simulink model "EGRVlv_VDMon_5818"  (R2016b)
settings: configuration reference "CodeGenConfigSet" (kept outside this file)
values from neighbouring files (symbols this model uses):
  EGRVlv_numLckdDetThres_C = Calibration.Parameter    [init_EGRVlv_VDMon.m]    (also in init_EGRVlv_VDMon_SIL.m = Simulink.Parameter)
  EGRVlv_numMonEngTemp_C = Calibration.Parameter    [init_EGRVlv_VDMon.m]    (also in init_EGRVlv_VDMon_SIL.m = Simulink.Parameter)
  EGRVlv_rDvtMax_C = Calibration.Parameter    [init_EGRVlv_VDMon.m]    (also in init_EGRVlv_VDMon_SIL.m = Simulink.Parameter)
  EGRVlv_rDvtMin_C = Calibration.Parameter    [init_EGRVlv_VDMon.m]    (also in init_EGRVlv_VDMon_SIL.m = Simulink.Parameter)
  EGRVlv_rJamVlvOpnDemMax_C = Calibration.Parameter    [init_EGRVlv_VDMon.m]    (also in init_EGRVlv_VDMon_SIL.m = Simulink.Parameter)
  EGRVlv_rJamVlvOpnHi_C = Calibration.Parameter    [init_EGRVlv_VDMon.m]    (also in init_EGRVlv_VDMon_SIL.m = Simulink.Parameter)
  EGRVlv_rJamVlvOpnLo_C = Calibration.Parameter    [init_EGRVlv_VDMon.m]    (also in init_EGRVlv_VDMon_SIL.m = Simulink.Parameter)
  EGRVlv_rLckdDetThres_C = Calibration.Parameter    [init_EGRVlv_VDMon.m]    (also in init_EGRVlv_VDMon_SIL.m = Simulink.Parameter)
  EGRVlv_rLMSActPosThresInit_C = Calibration.Parameter    [init_EGRVlv_VDMon.m]    (also in init_EGRVlv_VDMon_SIL.m = Simulink.Parameter)
  EGRVlv_rLMSActThresDwn_C = Calibration.Parameter    [init_EGRVlv_VDMon.m]    (also in init_EGRVlv_VDMon_SIL.m = Simulink.Parameter)
  EGRVlv_rLMSThresDwn_C = Calibration.Parameter    [init_EGRVlv_VDMon.m]    (also in init_EGRVlv_VDMon_SIL.m = Simulink.Parameter)
  EGRVlv_rLMSThresUp_C = Calibration.Parameter    [init_EGRVlv_VDMon.m]    (also in init_EGRVlv_VDMon_SIL.m = Simulink.Parameter)
  EGRVlv_RlsIKi_C = Calibration.Parameter    [init_EGRVlv_VDMon.m]    (also in init_EGRVlv_VDMon_SIL.m = Simulink.Parameter)
  EGRVlv_rRlsMax_C = Calibration.Parameter    [init_EGRVlv_VDMon.m]    (also in init_EGRVlv_VDMon_SIL.m = Simulink.Parameter)
  EGRVlv_rStpThres_C = Calibration.Parameter    [init_EGRVlv_VDMon.m]    (also in init_EGRVlv_VDMon_SIL.m = Simulink.Parameter)
  EGRVlv_swtGovByp_C = Calibration.Parameter    [init_EGRVlv_VDMon.m]    (also in init_EGRVlv_VDMon_SIL.m = Simulink.Parameter)
  EGRVlv_tEngHi_C = Calibration.Parameter    [init_EGRVlv_VDMon.m]    (also in init_EGRVlv_VDMon_SIL.m = Simulink.Parameter)
  EGRVlv_tEngLo_C = Calibration.Parameter    [init_EGRVlv_VDMon.m]    (also in init_EGRVlv_VDMon_SIL.m = Simulink.Parameter)
  EGRVlv_tiGovDvtMaxDebDef_C = Calibration.Parameter    [init_EGRVlv_VDMon.m]    (also in init_EGRVlv_VDMon_SIL.m = Simulink.Parameter)
  EGRVlv_tiGovDvtMaxDebOk_C = Calibration.Parameter    [init_EGRVlv_VDMon.m]    (also in init_EGRVlv_VDMon_SIL.m = Simulink.Parameter)
  EGRVlv_tiGovDvtMinDebDef_C = Calibration.Parameter    [init_EGRVlv_VDMon.m]    (also in init_EGRVlv_VDMon_SIL.m = Simulink.Parameter)
  EGRVlv_tiGovDvtMinDebOk_C = Calibration.Parameter    [init_EGRVlv_VDMon.m]    (also in init_EGRVlv_VDMon_SIL.m = Simulink.Parameter)
  EGRVlv_tiLMS_C = Calibration.Parameter    [init_EGRVlv_VDMon.m]    (also in init_EGRVlv_VDMon_SIL.m = Simulink.Parameter)
  EGRVlv_tiRepRls_C = Calibration.Parameter    [init_EGRVlv_VDMon.m]    (also in init_EGRVlv_VDMon_SIL.m = Simulink.Parameter)
  EGRVlv_tiRls_C = Calibration.Parameter    [init_EGRVlv_VDMon.m]    (also in init_EGRVlv_VDMon_SIL.m = Simulink.Parameter)
undefined symbols (not defined in the file or in its folder): EGRVlv_VDMon_DT, EngState_conv
libraries: CXLib x25, simulink x14
settings Model: Creator=lvzhanghui  LastModifiedBy=zhulinfeng
settings ConfigSetRef: SourceLocation=Base Workspace

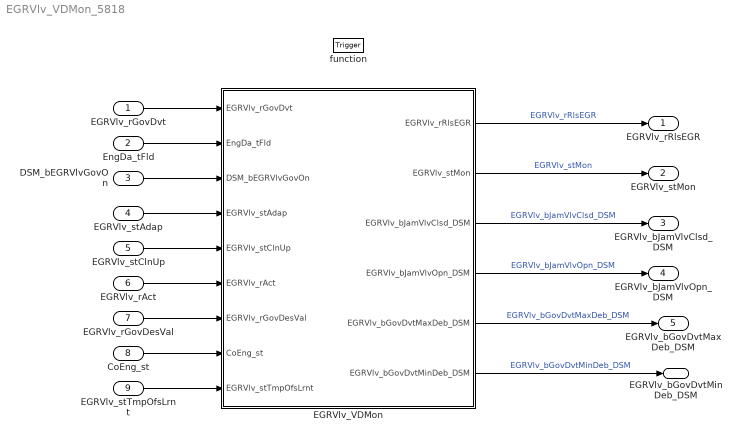
== system EGRVlv_VDMon_5818 ==
  EGRVlv_rGovDvt : Inport  Tag=%  Description=Control deviation  OutMin=-100  OutMax=100  OutDataTypeStr=Prc_100_rate
  EngDa_tFld : Inport  Tag=deg  Description=Engine temperature field  Port=2  OutMin=-3000  OutMax=3000  OutDataTypeStr=Temp_deg  PortDimensions=3
  DSM_bEGRVlvGovOn : Inport  Description=Status of FId_EGRVlvGovOn  Port=3  OutMin=0  OutMax=1  OutDataTypeStr=boolean
  EGRVlv_stAdap : Inport  Description=Status of offset learning  Port=4  OutMin=0  OutMax=65535  OutDataTypeStr=State_uint16
  EGRVlv_stClnUp : Inport  Description=Status of valvle cleanup function  Port=5  OutMin=0  OutMax=255  OutDataTypeStr=State_uint8
  EGRVlv_rAct : Inport  Tag=%  Description=Actuatorposition  Port=6  OutMin=-100  OutMax=100  OutDataTypeStr=Prc_100_rate
  EGRVlv_rGovDesVal : Inport  Tag=%  Description=Internal desired value for governor  Port=7  OutMin=-100  OutMax=100  OutDataTypeStr=Prc_100_rate
  CoEng_st : Inport  Description=Engine coordinator state  Port=8  OutDataTypeStr=Enum: EngState_conv
  EGRVlv_stTmpOfsLrnt : Inport  Description=Temporary offset of the EGR valve is already learnt in the current driving cycle  Port=9  OutMin=0  OutMax=1  OutDataTypeStr=boolean
  function : TriggerPort  TriggerType=function-call  VariantControl=Variant
  EGRVlv_VDMon : Subsystem
  EGRVlv_rRlsEGR : Outport  Tag=%  Description=Additional control value to release a jammed valve  OutMin=-100  OutMax=100  OutDataTypeStr=Prc_100_rate
  EGRVlv_stMon : Outport  Description=State of system monitoring  Port=2  OutMin=0  OutMax=65535  OutDataTypeStr=State_uint16
  EGRVlv_bJamVlvClsd_DSM : Outport  Description=Status of EGRVlv_bJamVlvClsd  Port=3  OutMin=0  OutMax=1  OutDataTypeStr=boolean
  EGRVlv_bJamVlvOpn_DSM : Outport  Description=Status of EGRVlv_bJamVlvOpn  Port=4  OutMin=0  OutMax=1  OutDataTypeStr=boolean
  EGRVlv_bGovDvtMaxDeb_DSM : Outport  Description=Status of EGRVlv_bGovDvtMaxDeb  Port=5  OutMin=0  OutMax=1  OutDataTypeStr=boolean
  EGRVlv_bGovDvtMinDeb_DSM : Outport  Description=Status of EGRVlv_bGovDvtMinDeb  Port=6  OutMin=0  OutMax=1  OutDataTypeStr=boolean
  wires:
  EGRVlv_rGovDvt/1 -> EGRVlv_VDMon/1(EGRVlv_rGovDvt)
  EngDa_tFld/1 -> EGRVlv_VDMon/2(EngDa_tFld)
  DSM_bEGRVlvGovOn/1 -> EGRVlv_VDMon/3(DSM_bEGRVlvGovOn)
  EGRVlv_stAdap/1 -> EGRVlv_VDMon/4(EGRVlv_stAdap)
  EGRVlv_stClnUp/1 -> EGRVlv_VDMon/5(EGRVlv_stClnUp)
  EGRVlv_rAct/1 -> EGRVlv_VDMon/6(EGRVlv_rAct)
  EGRVlv_rGovDesVal/1 -> EGRVlv_VDMon/7(EGRVlv_rGovDesVal)
  CoEng_st/1 -> EGRVlv_VDMon/8(CoEng_st)
  EGRVlv_stTmpOfsLrnt/1 -> EGRVlv_VDMon/9(EGRVlv_stTmpOfsLrnt)
  EGRVlv_VDMon/1(EGRVlv_rRlsEGR) -> EGRVlv_rRlsEGR/1  "EGRVlv_rRlsEGR"
  EGRVlv_VDMon/2(EGRVlv_stMon) -> EGRVlv_stMon/1  "EGRVlv_stMon"
  EGRVlv_VDMon/3(EGRVlv_bJamVlvClsd_DSM) -> EGRVlv_bJamVlvClsd_DSM/1  "EGRVlv_bJamVlvClsd_DSM"
  EGRVlv_VDMon/4(EGRVlv_bJamVlvOpn_DSM) -> EGRVlv_bJamVlvOpn_DSM/1  "EGRVlv_bJamVlvOpn_DSM"
  EGRVlv_VDMon/6(EGRVlv_bGovDvtMinDeb_DSM) -> EGRVlv_bGovDvtMinDeb_DSM/1  "EGRVlv_bGovDvtMinDeb_DSM"
  EGRVlv_VDMon/5(EGRVlv_bGovDvtMaxDeb_DSM) -> EGRVlv_bGovDvtMaxDeb_DSM/1  "EGRVlv_bGovDvtMaxDeb_DSM"

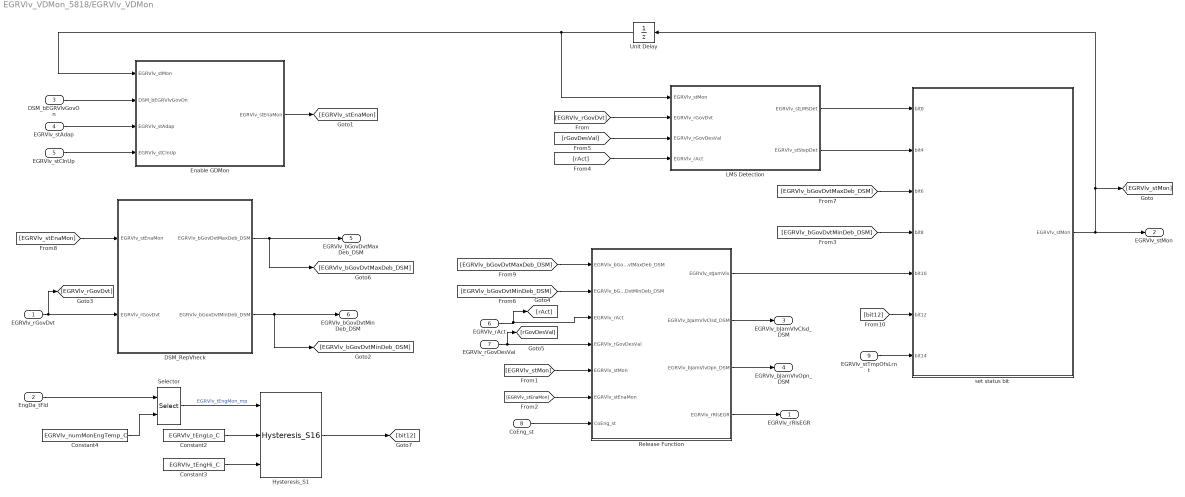
== system EGRVlv_VDMon_5818/EGRVlv_VDMon ==
  EGRVlv_rGovDvt : Inport  Tag=%
  EngDa_tFld : Inport  Tag=%  Port=2
  DSM_bEGRVlvGovOn : Inport  Tag=%  Port=3
  EGRVlv_stAdap : Inport  Tag=%  Port=4
  EGRVlv_stClnUp : Inport  Tag=%  Port=5
  EGRVlv_rAct : Inport  Tag=%  Port=6
  EGRVlv_rGovDesVal : Inport  Tag=%  Port=7
  CoEng_st : Inport  Tag=%  Port=8
  EGRVlv_stTmpOfsLrnt : Inport  Tag=%  Port=9
  Constant2 : Constant  Value=EGRVlv_tEngLo_C  SampleTime=-1
  Constant3 : Constant  Value=EGRVlv_tEngHi_C  SampleTime=-1
  Constant4 : Constant  Value=EGRVlv_numMonEngTemp_C  SampleTime=-1
  DSM_RepVheck : Subsystem
  Enable GDMon : Subsystem
  Hysteresis_S1 : CXLib/Hysteresis_S16
  LMS Detection : Subsystem
  Release Function : Subsystem
  Selector : Selector  IndexMode=Zero-based  InputPortWidth=3  IndexOptions=Index vector (port)  Indices=[1 3]  OutputSizes=1
  Unit Delay : UnitDelay  SampleTime=-1
      settings: AttributesFormatString=InitialValue=%<InitialCondition>
  set status bit : Subsystem
  EGRVlv_rRlsEGR : Outport  Tag=%
  EGRVlv_stMon : Outport  Tag=%  Port=2
  EGRVlv_bJamVlvClsd_DSM : Outport  Tag=%  Port=3
  EGRVlv_bJamVlvOpn_DSM : Outport  Tag=%  Port=4
  EGRVlv_bGovDvtMaxDeb_DSM : Outport  Description=Status of EGRVlv_bGovDvtMaxDeb  Port=5  OutMin=0  OutMax=1  OutDataTypeStr=boolean
  EGRVlv_bGovDvtMinDeb_DSM : Outport  Description=Status of EGRVlv_bGovDvtMinDeb  Port=6  OutMin=0  OutMax=1  OutDataTypeStr=boolean
  wires:
  Selector/1 -> Hysteresis_S1/1  "EGRVlv_tEngMon_mp"
  Release Function/1(EGRVlv_stJamVlv) -> set status bit/5(bit10)
  set status bit/1(EGRVlv_stMon) -> Unit Delay/1, [EGRVlv_stMon], EGRVlv_stMon/1
  Constant2/1 -> Hysteresis_S1/2
  DSM_RepVheck/2(EGRVlv_bGovDvtMinDeb_DSM) -> [EGRVlv_bGovDvtMinDeb_DSM], EGRVlv_bGovDvtMinDeb_DSM/1
  Constant3/1 -> Hysteresis_S1/3
  DSM_RepVheck/1(EGRVlv_bGovDvtMaxDeb_DSM) -> [EGRVlv_bGovDvtMaxDeb_DSM], EGRVlv_bGovDvtMaxDeb_DSM/1
  Constant4/1 -> Selector/2
  EngDa_tFld/1 -> Selector/1
  EGRVlv_rGovDvt/1 -> [EGRVlv_rGovDvt], DSM_RepVheck/2(EGRVlv_rGovDvt)
  EGRVlv_rAct/1 -> [rAct], Release Function/3(EGRVlv_rAct)
  EGRVlv_rGovDesVal/1 -> [rGovDesVal], Release Function/4(EGRVlv_rGovDesVal)
  Unit Delay/1 -> Enable GDMon/1(EGRVlv_stMon), LMS Detection/1(EGRVlv_stMon)
  LMS Detection/2(EGRVlv_stStepDet) -> set status bit/2(bit4)
  LMS Detection/1(EGRVlv_stLMSDet) -> set status bit/1(bit0)
  Enable GDMon/1(EGRVlv_stEnaMon) -> [EGRVlv_stEnaMon]
  DSM_bEGRVlvGovOn/1 -> Enable GDMon/2(DSM_bEGRVlvGovOn)
  EGRVlv_stAdap/1 -> Enable GDMon/3(EGRVlv_stAdap)
  EGRVlv_stClnUp/1 -> Enable GDMon/4(EGRVlv_stClnUp)
  [EGRVlv_rGovDvt] -> LMS Detection/2(EGRVlv_rGovDvt)
  [rGovDesVal] -> LMS Detection/3(EGRVlv_rGovDesVal)
  [rAct] -> LMS Detection/4(EGRVlv_rAct)
  [EGRVlv_stMon] -> Release Function/5(EGRVlv_stMon)
  [EGRVlv_stEnaMon] -> Release Function/6(EGRVlv_stEnaMon)
  CoEng_st/1 -> Release Function/7(CoEng_st)
  [EGRVlv_bGovDvtMinDeb_DSM] -> set status bit/4(bit8)
  EGRVlv_stTmpOfsLrnt/1 -> set status bit/7(bit14)
  Release Function/2(EGRVlv_bJamVlvClsd_DSM) -> EGRVlv_bJamVlvClsd_DSM/1
  Release Function/3(EGRVlv_bJamVlvOpn_DSM) -> EGRVlv_bJamVlvOpn_DSM/1
  Release Function/4(EGRVlv_rRlsEGR) -> EGRVlv_rRlsEGR/1
  [EGRVlv_bGovDvtMinDeb_DSM] -> Release Function/2(EGRVlv_bGovDvtMinDeb_DSM)
  [EGRVlv_bGovDvtMaxDeb_DSM] -> set status bit/3(bit6)
  [EGRVlv_stEnaMon] -> DSM_RepVheck/1(EGRVlv_stEnaMon)
  [EGRVlv_bGovDvtMaxDeb_DSM] -> Release Function/1(EGRVlv_bGovDvtMaxDeb_DSM)
  Hysteresis_S1/1 -> [bit12]
  [bit12] -> set status bit/6(bit12)

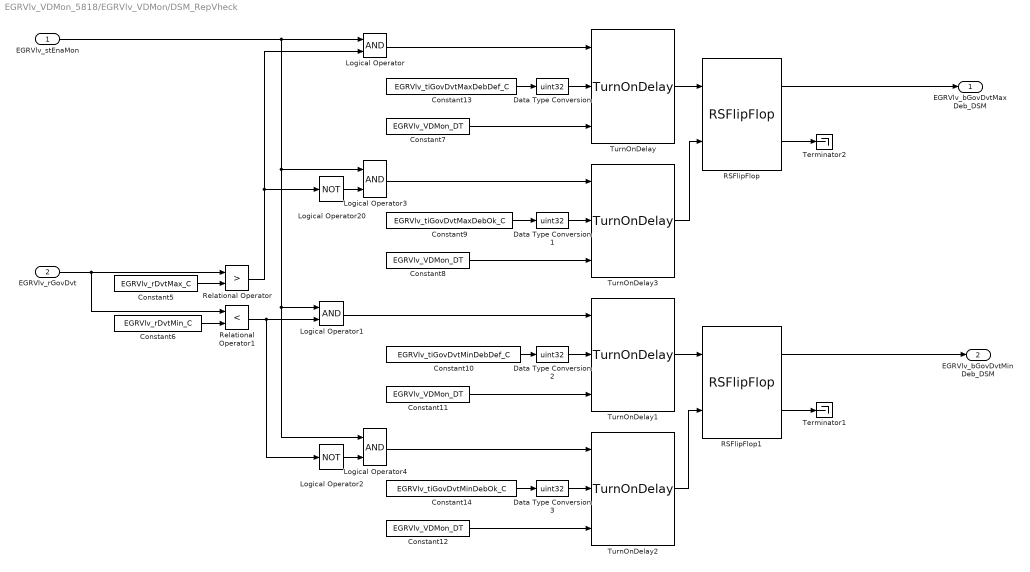
== system EGRVlv_VDMon_5818/EGRVlv_VDMon/DSM_RepVheck ==
  EGRVlv_stEnaMon : Inport  Tag=%
  EGRVlv_rGovDvt : Inport  Tag=%  Port=2
  Constant10 : Constant  Value=EGRVlv_tiGovDvtMinDebDef_C
  Constant{7..8,11..12} (4 alike) : Constant  Value=EGRVlv_VDMon_DT
  Constant13 : Constant  Value=EGRVlv_tiGovDvtMaxDebDef_C
  Constant14 : Constant  Value=EGRVlv_tiGovDvtMinDebOk_C
  Constant5 : Constant  Value=EGRVlv_rDvtMax_C  SampleTime=-1
  Constant6 : Constant  Value=EGRVlv_rDvtMin_C  SampleTime=-1
  Constant9 : Constant  Value=EGRVlv_tiGovDvtMaxDebOk_C
  Data Type Conversion{,1..3} (4 alike) : DataTypeConversion  OutDataTypeStr=uint32
  Logical Operator{,1,3..4} (4 alike) : Logic  AllPortsSameDT=off  OutDataTypeStr=boolean
  Logical Operator2 : Logic  Operator=NOT  AllPortsSameDT=off  OutDataTypeStr=boolean
  Logical Operator20 : Logic  Operator=NOT  AllPortsSameDT=off  OutDataTypeStr=boolean
  RSFlipFlop : CXLib/RSFlipFlop
  RSFlipFlop1 : CXLib/RSFlipFlop
  Relational Operator : RelationalOperator  Operator=>  OutDataTypeStr=boolean  RndMeth=Simplest
  Relational Operator1 : RelationalOperator  Operator=<  OutDataTypeStr=boolean  RndMeth=Simplest
  Terminator1 : Terminator
  Terminator2 : Terminator
  TurnOnDelay{,1..3} (4 alike) : CXLib/TurnOnDelay
  EGRVlv_bGovDvtMaxDeb_DSM : Outport  Tag=%
  EGRVlv_bGovDvtMinDeb_DSM : Outport  Tag=%  Port=2
  wires:
  Constant9/1 -> Data Type Conversion1/1
  Constant12/1 -> TurnOnDelay2/3
  Logical Operator/1 -> TurnOnDelay/1
  Constant10/1 -> Data Type Conversion2/1
  TurnOnDelay2/1 -> RSFlipFlop1/2
  TurnOnDelay1/1 -> RSFlipFlop1/1
  Constant8/1 -> TurnOnDelay3/3
  Relational Operator1/1 -> Logical Operator2/1, Logical Operator1/2
  Constant11/1 -> TurnOnDelay1/3
  EGRVlv_rGovDvt/1 -> Relational Operator/1, Relational Operator1/1
  Relational Operator/1 -> Logical Operator/2, Logical Operator20/1
  Constant6/1 -> Relational Operator1/2
  Logical Operator1/1 -> TurnOnDelay1/1
  Constant13/1 -> Data Type Conversion/1
  TurnOnDelay3/1 -> RSFlipFlop/2
  Constant7/1 -> TurnOnDelay/3
  Constant14/1 -> Data Type Conversion3/1
  Constant5/1 -> Relational Operator/2
  TurnOnDelay/1 -> RSFlipFlop/1
  EGRVlv_stEnaMon/1 -> Logical Operator3/1, Logical Operator4/1, Logical Operator1/1, Logical Operator/1
  Data Type Conversion/1 -> TurnOnDelay/2
  Data Type Conversion1/1 -> TurnOnDelay3/2
  Data Type Conversion2/1 -> TurnOnDelay1/2
  Data Type Conversion3/1 -> TurnOnDelay2/2
  Logical Operator20/1 -> Logical Operator3/2
  Logical Operator3/1 -> TurnOnDelay3/1
  Logical Operator2/1 -> Logical Operator4/2
  Logical Operator4/1 -> TurnOnDelay2/1
  RSFlipFlop1/1 -> EGRVlv_bGovDvtMinDeb_DSM/1
  RSFlipFlop1/2 -> Terminator1/1
  RSFlipFlop/1 -> EGRVlv_bGovDvtMaxDeb_DSM/1
  RSFlipFlop/2 -> Terminator2/1

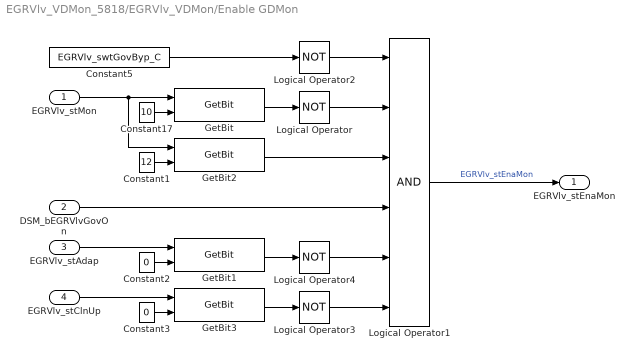
== system EGRVlv_VDMon_5818/EGRVlv_VDMon/Enable GDMon ==
  EGRVlv_stMon : Inport  Tag=%
  DSM_bEGRVlvGovOn : Inport  Tag=%  Port=2
  EGRVlv_stAdap : Inport  Tag=%  Port=3
  EGRVlv_stClnUp : Inport  Tag=%  Port=4
  Constant1 : Constant  Value=12  OutDataTypeStr=uint8
  Constant17 : Constant  Value=10  OutDataTypeStr=uint8
  Constant2 : Constant  Value=0  OutDataTypeStr=uint8
  Constant3 : Constant  Value=0  OutDataTypeStr=uint8
  Constant5 : Constant  Value=EGRVlv_swtGovByp_C  SampleTime=-1
  GetBit : CXLib/GetBit  dataTypeString=uint16  dataLength=0
      settings: AttributesFormatString=Get bit from %<dataTypeString>
  GetBit1 : CXLib/GetBit  dataTypeString=uint16  dataLength=0
      settings: AttributesFormatString=Get bit from %<dataTypeString>
  GetBit2 : CXLib/GetBit  dataTypeString=uint16  dataLength=0
      settings: AttributesFormatString=Get bit from %<dataTypeString>
  GetBit3 : CXLib/GetBit  dataTypeString=uint8  dataLength=0
      settings: AttributesFormatString=Get bit from %<dataTypeString>
  Logical Operator{,2..4} (4 alike) : Logic  Operator=NOT  AllPortsSameDT=off  OutDataTypeStr=boolean
  Logical Operator1 : Logic  Inputs=6  AllPortsSameDT=off  OutDataTypeStr=boolean
  EGRVlv_stEnaMon : Outport  Tag=%
  wires:
  Logical Operator/1 -> Logical Operator1/2
  Constant5/1 -> Logical Operator2/1
  GetBit2/1 -> Logical Operator1/3
  GetBit1/1 -> Logical Operator4/1
  Logical Operator3/1 -> Logical Operator1/6
  GetBit3/1 -> Logical Operator3/1
  Logical Operator4/1 -> Logical Operator1/5
  Logical Operator1/1 -> EGRVlv_stEnaMon/1  "EGRVlv_stEnaMon"
  Logical Operator2/1 -> Logical Operator1/1
  DSM_bEGRVlvGovOn/1 -> Logical Operator1/4
  GetBit/1 -> Logical Operator/1
  Constant17/1 -> GetBit/2
  Constant1/1 -> GetBit2/2
  Constant2/1 -> GetBit1/2
  Constant3/1 -> GetBit3/2
  EGRVlv_stMon/1 -> GetBit2/1, GetBit/1
  EGRVlv_stAdap/1 -> GetBit1/1
  EGRVlv_stClnUp/1 -> GetBit3/1

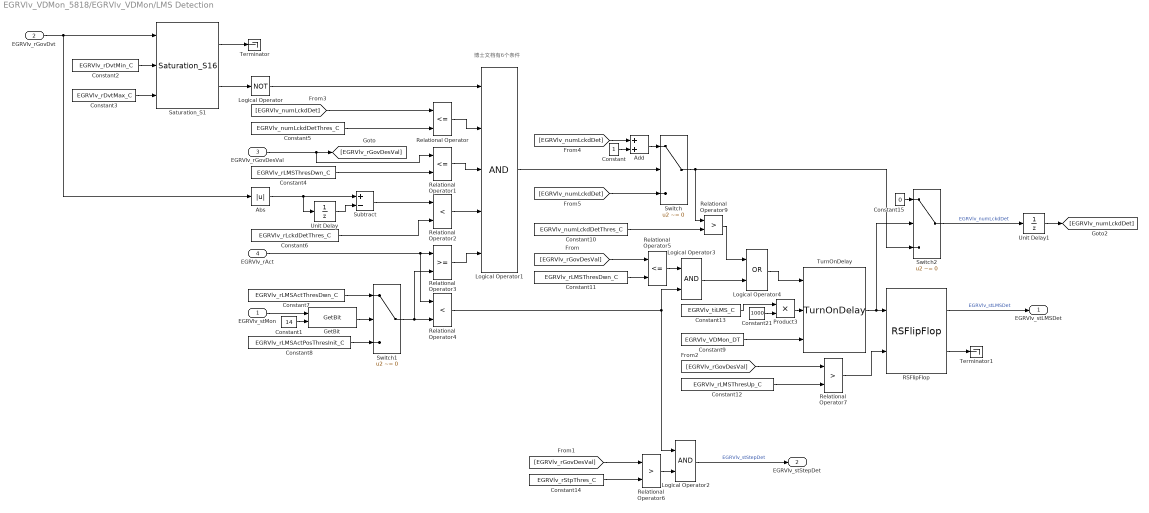
== system EGRVlv_VDMon_5818/EGRVlv_VDMon/LMS Detection ==
  note: 博士文档有6个条件
  EGRVlv_stMon : Inport  Tag=%
  EGRVlv_rGovDvt : Inport  Tag=%  Port=2
  EGRVlv_rGovDesVal : Inport  Tag=%  Port=3
  EGRVlv_rAct : Inport  Tag=%  Port=4
  Abs : Abs
  Add : Sum  SaturateOnIntegerOverflow=on
  Constant : Constant  OutDataTypeStr=Inherit: Inherit via back propagation
  Constant1 : Constant  Value=14  OutDataTypeStr=uint8
  Constant10 : Constant  Value=EGRVlv_numLckdDetThres_C
  Constant11 : Constant  Value=EGRVlv_rLMSThresDwn_C
  Constant12 : Constant  Value=EGRVlv_rLMSThresUp_C
  Constant13 : Constant  Value=EGRVlv_tiLMS_C
  Constant14 : Constant  Value=EGRVlv_rStpThres_C
  Constant15 : Constant  Value=0  OutDataTypeStr=Inherit: Inherit via back propagation
  Constant2 : Constant  Value=EGRVlv_rDvtMin_C  SampleTime=-1
  Constant21 : Constant  Value=1000  OutDataTypeStr=uint16
  Constant3 : Constant  Value=EGRVlv_rDvtMax_C  SampleTime=-1
  Constant4 : Constant  Value=EGRVlv_rLMSThresDwn_C  SampleTime=-1
  Constant5 : Constant  Value=EGRVlv_numLckdDetThres_C  SampleTime=-1
  Constant6 : Constant  Value=EGRVlv_rLckdDetThres_C  SampleTime=-1
  Constant7 : Constant  Value=EGRVlv_rLMSActThresDwn_C  SampleTime=-1
  Constant8 : Constant  Value=EGRVlv_rLMSActPosThresInit_C  SampleTime=-1
  Constant9 : Constant  Value=EGRVlv_VDMon_DT
  GetBit : CXLib/GetBit  dataTypeString=uint16  dataLength=0
      settings: AttributesFormatString=Get bit from %<dataTypeString>
  Logical Operator : Logic  Operator=NOT  AllPortsSameDT=off  OutDataTypeStr=boolean
  Logical Operator1 : Logic  Inputs=5  AllPortsSameDT=off  OutDataTypeStr=boolean
  Logical Operator2 : Logic  AllPortsSameDT=off  OutDataTypeStr=boolean
  Logical Operator3 : Logic  AllPortsSameDT=off  OutDataTypeStr=boolean
  Logical Operator4 : Logic  Operator=OR  AllPortsSameDT=off  OutDataTypeStr=boolean
  Product3 : Product  OutDataTypeStr=uint32  SaturateOnIntegerOverflow=on
  RSFlipFlop : CXLib/RSFlipFlop
  Relational Operator : RelationalOperator  Operator=<=  OutDataTypeStr=boolean  RndMeth=Simplest
  Relational Operator1 : RelationalOperator  Operator=<=  OutDataTypeStr=boolean  RndMeth=Simplest
  Relational Operator2 : RelationalOperator  Operator=<  OutDataTypeStr=boolean  RndMeth=Simplest
  Relational Operator3 : RelationalOperator  OutDataTypeStr=boolean  RndMeth=Simplest
  Relational Operator4 : RelationalOperator  Operator=<  OutDataTypeStr=boolean  RndMeth=Simplest
  Relational Operator5 : RelationalOperator  Operator=<=  OutDataTypeStr=boolean  RndMeth=Simplest
  Relational Operator6 : RelationalOperator  Operator=>  OutDataTypeStr=boolean  RndMeth=Simplest
  Relational Operator7 : RelationalOperator  Operator=>  OutDataTypeStr=boolean  RndMeth=Simplest
  Relational Operator9 : RelationalOperator  Operator=>  OutDataTypeStr=boolean  RndMeth=Simplest
  Saturation_S1 : CXLib/Saturation_S16
  Subtract : Sum  Inputs=+-  SaturateOnIntegerOverflow=on
  Switch : Switch  Criteria=u2 ~= 0
  Switch1 : Switch  Criteria=u2 ~= 0
  Switch2 : Switch  Criteria=u2 ~= 0
  Terminator : Terminator
  Terminator1 : Terminator
  TurnOnDelay : CXLib/TurnOnDelay
  Unit Delay : UnitDelay  SampleTime=-1
      settings: AttributesFormatString=InitialValue=%<InitialCondition>
  Unit Delay1 : UnitDelay  SampleTime=-1
      settings: AttributesFormatString=InitialValue=%<InitialCondition>
  EGRVlv_stLMSDet : Outport  Tag=%
  EGRVlv_stStepDet : Outport  Tag=%  Port=2
  wires:
  Saturation_S1/2 -> Logical Operator/1
  Constant1/1 -> GetBit/2
  Relational Operator/1 -> Logical Operator1/2
  Relational Operator1/1 -> Logical Operator1/3
  Relational Operator2/1 -> Logical Operator1/4
  Relational Operator3/1 -> Logical Operator1/5
  Constant5/1 -> Relational Operator/2
  Constant2/1 -> Saturation_S1/2
  Constant3/1 -> Saturation_S1/3
  EGRVlv_rGovDvt/1 -> Saturation_S1/1, Abs/1
  [EGRVlv_numLckdDet] -> Relational Operator/1
  Constant4/1 -> Relational Operator1/2
  EGRVlv_rGovDesVal/1 -> [EGRVlv_rGovDesVal], Relational Operator1/1
  Subtract/1 -> Relational Operator2/1
  Abs/1 -> Unit Delay/1, Subtract/1
  Unit Delay/1 -> Subtract/2
  Constant6/1 -> Relational Operator2/2
  Logical Operator1/1 -> Switch/2
  Add/1 -> Switch/1
  Constant/1 -> Add/2
  Constant7/1 -> Switch1/1
  Constant8/1 -> Switch1/3
  GetBit/1 -> Switch1/2
  Switch1/1 -> Relational Operator3/2, Relational Operator4/2
  Relational Operator6/1 -> Logical Operator2/2
  Relational Operator4/1 -> Logical Operator2/1, Logical Operator3/2
  Relational Operator5/1 -> Logical Operator3/1
  Logical Operator3/1 -> Logical Operator4/2
  Relational Operator9/1 -> Logical Operator4/1
  Constant9/1 -> TurnOnDelay/3
  TurnOnDelay/1 -> RSFlipFlop/1, Switch2/2
  Logical Operator4/1 -> TurnOnDelay/1
  Relational Operator7/1 -> RSFlipFlop/2
  Constant10/1 -> Relational Operator9/2
  [EGRVlv_rGovDesVal] -> Relational Operator5/1
  Constant11/1 -> Relational Operator5/2
  Constant12/1 -> Relational Operator7/2
  Constant14/1 -> Relational Operator6/2
  [EGRVlv_rGovDesVal] -> Relational Operator7/1
  Logical Operator2/1 -> EGRVlv_stStepDet/1  "EGRVlv_stStepDet"
  EGRVlv_rAct/1 -> Relational Operator4/1, Relational Operator3/1
  Constant15/1 -> Switch2/1
  Switch2/1 -> Unit Delay1/1  "EGRVlv_numLckdDet"
  Unit Delay1/1 -> [EGRVlv_numLckdDet]
  [EGRVlv_numLckdDet] -> Add/1
  [EGRVlv_numLckdDet] -> Switch/3
  Switch/1 -> Relational Operator9/1, Switch2/3
  [EGRVlv_rGovDesVal] -> Relational Operator6/1
  Logical Operator/1 -> Logical Operator1/1
  Constant21/1 -> Product3/2
  Constant13/1 -> Product3/1
  Product3/1 -> TurnOnDelay/2
  EGRVlv_stMon/1 -> GetBit/1
  RSFlipFlop/1 -> EGRVlv_stLMSDet/1  "EGRVlv_stLMSDet"
  RSFlipFlop/2 -> Terminator1/1
  Saturation_S1/1 -> Terminator/1

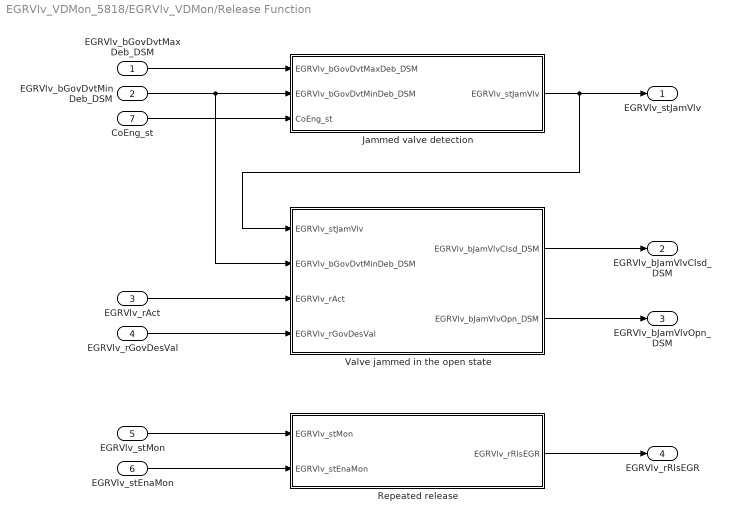
== system EGRVlv_VDMon_5818/EGRVlv_VDMon/Release Function ==
  EGRVlv_bGovDvtMaxDeb_DSM : Inport  Tag=%
  EGRVlv_bGovDvtMinDeb_DSM : Inport  Tag=%  Port=2
  EGRVlv_rAct : Inport  Tag=%  Port=3
  EGRVlv_rGovDesVal : Inport  Tag=%  Port=4
  EGRVlv_stMon : Inport  Tag=%  Port=5
  EGRVlv_stEnaMon : Inport  Tag=%  Port=6
  CoEng_st : Inport  Tag=%  Port=7
  Jammed valve detection : Subsystem
  Repeated release : Subsystem
  Valve jammed in the open state : Subsystem
  EGRVlv_stJamVlv : Outport  Tag=%
  EGRVlv_bJamVlvClsd_DSM : Outport  Tag=%  Port=2
  EGRVlv_bJamVlvOpn_DSM : Outport  Tag=%  Port=3
  EGRVlv_rRlsEGR : Outport  Tag=%  Port=4
  wires:
  EGRVlv_bGovDvtMinDeb_DSM/1 -> Jammed valve detection/2(EGRVlv_bGovDvtMinDeb_DSM), Valve jammed in the open state/2(EGRVlv_bGovDvtMinDeb_DSM)
  Jammed valve detection/1(EGRVlv_stJamVlv) -> EGRVlv_stJamVlv/1, Valve jammed in the open state/1(EGRVlv_stJamVlv)
  EGRVlv_bGovDvtMaxDeb_DSM/1 -> Jammed valve detection/1(EGRVlv_bGovDvtMaxDeb_DSM)
  CoEng_st/1 -> Jammed valve detection/3(CoEng_st)
  EGRVlv_stMon/1 -> Repeated release/1(EGRVlv_stMon)
  EGRVlv_stEnaMon/1 -> Repeated release/2(EGRVlv_stEnaMon)
  EGRVlv_rAct/1 -> Valve jammed in the open state/3(EGRVlv_rAct)
  EGRVlv_rGovDesVal/1 -> Valve jammed in the open state/4(EGRVlv_rGovDesVal)
  Repeated release/1(EGRVlv_rRlsEGR) -> EGRVlv_rRlsEGR/1
  Valve jammed in the open state/1(EGRVlv_bJamVlvClsd_DSM) -> EGRVlv_bJamVlvClsd_DSM/1
  Valve jammed in the open state/2(EGRVlv_bJamVlvOpn_DSM) -> EGRVlv_bJamVlvOpn_DSM/1

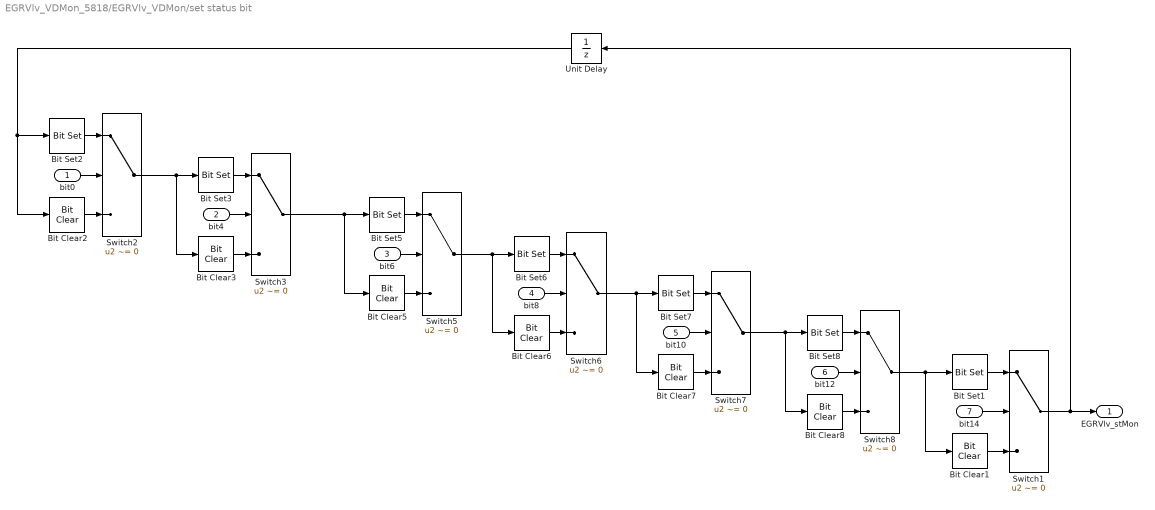
== system EGRVlv_VDMon_5818/EGRVlv_VDMon/set status bit ==
  bit0 : Inport
  bit4 : Inport  Port=2
  bit6 : Inport  Port=3
  bit8 : Inport  Port=4
  bit10 : Inport  Port=5
  bit12 : Inport  Port=6
  bit14 : Inport  Port=7
  Bit Clear1 : simulink/Logic and Bit Operations/Bit Clear  iBit=14
  Bit Clear2 : simulink/Logic and Bit Operations/Bit Clear  iBit=0
  Bit Clear3 : simulink/Logic and Bit Operations/Bit Clear  iBit=4
  Bit Clear5 : simulink/Logic and Bit Operations/Bit Clear  iBit=6
  Bit Clear6 : simulink/Logic and Bit Operations/Bit Clear  iBit=8
  Bit Clear7 : simulink/Logic and Bit Operations/Bit Clear  iBit=10
  Bit Clear8 : simulink/Logic and Bit Operations/Bit Clear  iBit=12
  Bit Set1 : simulink/Logic and Bit Operations/Bit Set  iBit=14
  Bit Set2 : simulink/Logic and Bit Operations/Bit Set  iBit=0
  Bit Set3 : simulink/Logic and Bit Operations/Bit Set  iBit=4
  Bit Set5 : simulink/Logic and Bit Operations/Bit Set  iBit=6
  Bit Set6 : simulink/Logic and Bit Operations/Bit Set  iBit=8
  Bit Set7 : simulink/Logic and Bit Operations/Bit Set  iBit=10
  Bit Set8 : simulink/Logic and Bit Operations/Bit Set  iBit=12
  Switch{1..3,5..8} (7 alike) : Switch  Criteria=u2 ~= 0  OutDataTypeStr=Inherit: Inherit via back propagation  SaturateOnIntegerOverflow=on  InputSameDT=on
  Unit Delay : UnitDelay  SampleTime=-1
      settings: AttributesFormatString=InitialValue=%<InitialCondition>
  EGRVlv_stMon : Outport
  wires:
  bit12/1 -> Switch8/2
  Switch7/1 -> Bit Clear8/1, Bit Set8/1
  Bit Clear8/1 -> Switch8/3
  Bit Set8/1 -> Switch8/1
  bit10/1 -> Switch7/2
  Switch6/1 -> Bit Set7/1, Bit Clear7/1
  Bit Clear7/1 -> Switch7/3
  Bit Set7/1 -> Switch7/1
  bit8/1 -> Switch6/2
  Switch5/1 -> Bit Clear6/1, Bit Set6/1
  Bit Clear6/1 -> Switch6/3
  Bit Set6/1 -> Switch6/1
  bit6/1 -> Switch5/2
  Bit Clear5/1 -> Switch5/3
  Bit Set5/1 -> Switch5/1
  bit14/1 -> Switch1/2
  Bit Clear1/1 -> Switch1/3
  Bit Set1/1 -> Switch1/1
  Switch1/1 -> Unit Delay/1, EGRVlv_stMon/1
  Switch8/1 -> Bit Clear1/1, Bit Set1/1
  bit4/1 -> Switch3/2
  Switch2/1 -> Bit Set3/1, Bit Clear3/1
  Bit Clear3/1 -> Switch3/3
  Bit Set3/1 -> Switch3/1
  bit0/1 -> Switch2/2
  Bit Clear2/1 -> Switch2/3
  Bit Set2/1 -> Switch2/1
  Switch3/1 -> Bit Clear5/1, Bit Set5/1
  Unit Delay/1 -> Bit Clear2/1, Bit Set2/1

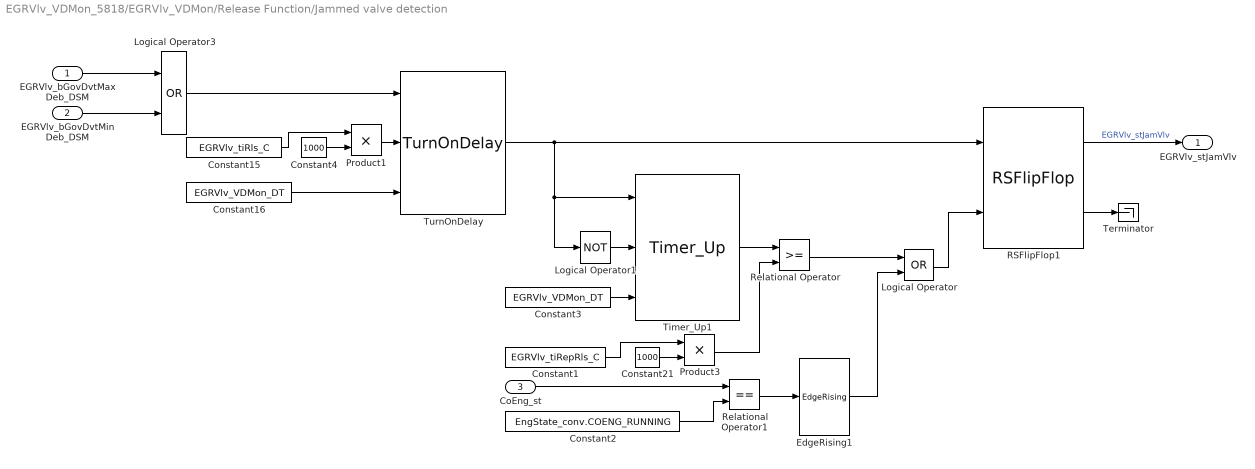
== system EGRVlv_VDMon_5818/EGRVlv_VDMon/Release Function/Jammed valve detection ==
  EGRVlv_bGovDvtMaxDeb_DSM : Inport  Tag=%
  EGRVlv_bGovDvtMinDeb_DSM : Inport  Tag=%  Port=2
  CoEng_st : Inport  Tag=%  Port=3
  Constant1 : Constant  Value=EGRVlv_tiRepRls_C
  Constant15 : Constant  Value=EGRVlv_tiRls_C
  Constant16 : Constant  Value=EGRVlv_VDMon_DT
  Constant2 : Constant  Value=EngState_conv.COENG_RUNNING
  Constant21 : Constant  Value=1000  OutDataTypeStr=uint16
  Constant3 : Constant  Value=EGRVlv_VDMon_DT
  Constant4 : Constant  Value=1000  OutDataTypeStr=uint16
  EdgeRising1 : CXLib/EdgeRising
  Logical Operator : Logic  Operator=OR  AllPortsSameDT=off  OutDataTypeStr=boolean
  Logical Operator1 : Logic  Operator=NOT  AllPortsSameDT=off  OutDataTypeStr=boolean
  Logical Operator3 : Logic  Operator=OR  AllPortsSameDT=off  OutDataTypeStr=boolean
  Product1 : Product  OutDataTypeStr=uint32  SaturateOnIntegerOverflow=on
  Product3 : Product  OutDataTypeStr=uint32  SaturateOnIntegerOverflow=on
  RSFlipFlop1 : CXLib/RSFlipFlop
  Relational Operator : RelationalOperator  OutDataTypeStr=boolean  RndMeth=Simplest
  Relational Operator1 : RelationalOperator  Operator===  OutDataTypeStr=boolean  RndMeth=Simplest
  Terminator : Terminator
  Timer_Up1 : CXLib/Timer_Up
  TurnOnDelay : CXLib/TurnOnDelay
  EGRVlv_stJamVlv : Outport  Tag=%
  wires:
  Logical Operator3/1 -> TurnOnDelay/1
  EGRVlv_bGovDvtMinDeb_DSM/1 -> Logical Operator3/2
  EGRVlv_bGovDvtMaxDeb_DSM/1 -> Logical Operator3/1
  TurnOnDelay/1 -> RSFlipFlop1/1, Timer_Up1/1, Logical Operator1/1
  Constant16/1 -> TurnOnDelay/3
  Timer_Up1/1 -> Relational Operator/1
  Relational Operator/1 -> Logical Operator/1
  CoEng_st/1 -> Relational Operator1/1
  Constant2/1 -> Relational Operator1/2
  Logical Operator/1 -> RSFlipFlop1/2
  Constant3/1 -> Timer_Up1/3
  Logical Operator1/1 -> Timer_Up1/2
  Relational Operator1/1 -> EdgeRising1/1
  EdgeRising1/1 -> Logical Operator/2
  Constant21/1 -> Product3/2
  Constant1/1 -> Product3/1
  Product3/1 -> Relational Operator/2
  Constant4/1 -> Product1/2
  Constant15/1 -> Product1/1
  Product1/1 -> TurnOnDelay/2
  RSFlipFlop1/1 -> EGRVlv_stJamVlv/1  "EGRVlv_stJamVlv"
  RSFlipFlop1/2 -> Terminator/1

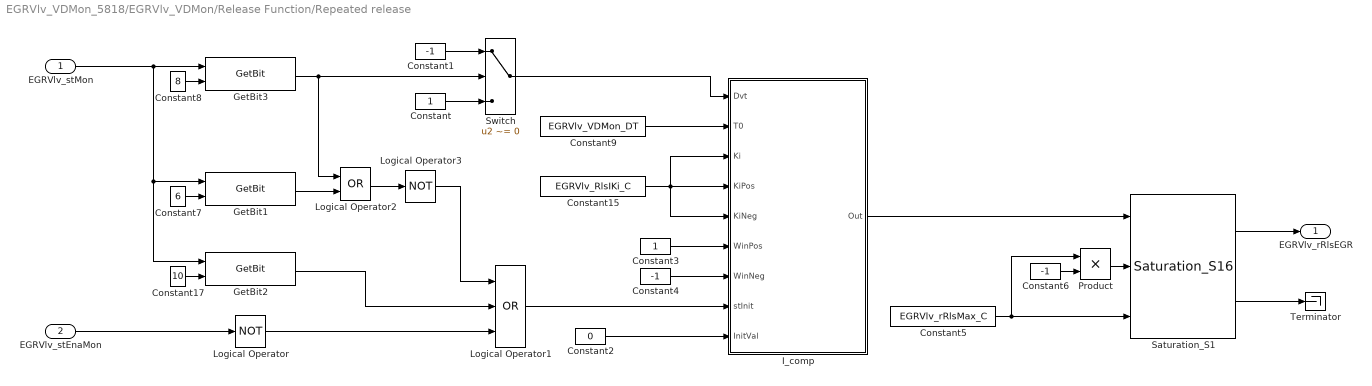
== system EGRVlv_VDMon_5818/EGRVlv_VDMon/Release Function/Repeated release ==
  EGRVlv_stMon : Inport  Tag=%
  EGRVlv_stEnaMon : Inport  Tag=%  Port=2
  Constant : Constant  OutMin=-100  OutMax=100  OutDataTypeStr=Prc_100_rate
  Constant1 : Constant  Value=-1  OutMin=-100  OutMax=100  OutDataTypeStr=Prc_100_rate
  Constant15 : Constant  Value=EGRVlv_RlsIKi_C
  Constant17 : Constant  Value=10  OutDataTypeStr=uint8
  Constant2 : Constant  Value=0  OutDataTypeStr=Prc_100_rate
  Constant3 : Constant  OutDataTypeStr=Prc_100_rate
  Constant4 : Constant  Value=-1  OutDataTypeStr=Prc_100_rate
  Constant5 : Constant  Value=EGRVlv_rRlsMax_C
  Constant6 : Constant  Value=-1  OutDataTypeStr=int8
  Constant7 : Constant  Value=6  OutDataTypeStr=uint8
  Constant8 : Constant  Value=8  OutDataTypeStr=uint8
  Constant9 : Constant  Value=EGRVlv_VDMon_DT
  GetBit1 : CXLib/GetBit  dataTypeString=uint16  dataLength=0
      settings: AttributesFormatString=Get bit from %<dataTypeString>
  GetBit2 : CXLib/GetBit  dataTypeString=uint16  dataLength=0
      settings: AttributesFormatString=Get bit from %<dataTypeString>
  GetBit3 : CXLib/GetBit  dataTypeString=uint16  dataLength=0
      settings: AttributesFormatString=Get bit from %<dataTypeString>
  I_comp : Subsystem
  Logical Operator : Logic  Operator=NOT  AllPortsSameDT=off  OutDataTypeStr=boolean
  Logical Operator1 : Logic  Operator=OR  Inputs=3  AllPortsSameDT=off  OutDataTypeStr=boolean
  Logical Operator2 : Logic  Operator=OR  AllPortsSameDT=off  OutDataTypeStr=boolean
  Logical Operator3 : Logic  Operator=NOT  AllPortsSameDT=off  OutDataTypeStr=boolean
  Product : Product  OutDataTypeStr=Prc_100_rate  SaturateOnIntegerOverflow=on
  Saturation_S1 : CXLib/Saturation_S16
  Switch : Switch  Criteria=u2 ~= 0
  Terminator : Terminator
  EGRVlv_rRlsEGR : Outport  Tag=%
  wires:
  Product/1 -> Saturation_S1/2
  Logical Operator3/1 -> Logical Operator1/1
  Constant1/1 -> Switch/1
  Logical Operator/1 -> Logical Operator1/3
  Constant/1 -> Switch/3
  EGRVlv_stEnaMon/1 -> Logical Operator/1
  GetBit3/1 -> Logical Operator2/1, Switch/2
  Switch/1 -> I_comp/1(Dvt)
  GetBit1/1 -> Logical Operator2/2
  Logical Operator2/1 -> Logical Operator3/1
  Constant6/1 -> Product/2
  GetBit2/1 -> Logical Operator1/2
  Constant5/1 -> Product/1, Saturation_S1/3
  I_comp/1(Out) -> Saturation_S1/1
  Constant15/1 -> I_comp/5(KiNeg), I_comp/3(Ki), I_comp/4(KiPos)
  Constant4/1 -> I_comp/7(WinNeg)
  Constant3/1 -> I_comp/6(WinPos)
  Constant17/1 -> GetBit2/2
  Constant7/1 -> GetBit1/2
  Constant8/1 -> GetBit3/2
  EGRVlv_stMon/1 -> GetBit3/1, GetBit2/1, GetBit1/1
  Saturation_S1/1 -> EGRVlv_rRlsEGR/1
  Saturation_S1/2 -> Terminator/1
  Constant2/1 -> I_comp/9(InitVal)
  Logical Operator1/1 -> I_comp/8(stInit)
  Constant9/1 -> I_comp/2(T0)

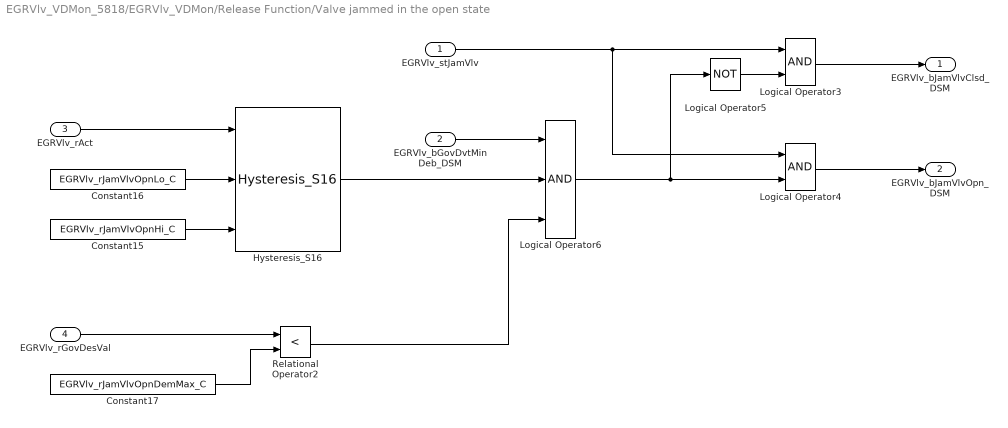
== system EGRVlv_VDMon_5818/EGRVlv_VDMon/Release Function/Valve jammed in the open state ==
  EGRVlv_stJamVlv : Inport  Tag=%
  EGRVlv_bGovDvtMinDeb_DSM : Inport  Tag=%  Port=2
  EGRVlv_rAct : Inport  Tag=%  Port=3
  EGRVlv_rGovDesVal : Inport  Tag=%  Port=4
  Constant15 : Constant  Value=EGRVlv_rJamVlvOpnHi_C
  Constant16 : Constant  Value=EGRVlv_rJamVlvOpnLo_C
  Constant17 : Constant  Value=EGRVlv_rJamVlvOpnDemMax_C
  Hysteresis_S16 : CXLib/Hysteresis_S16
  Logical Operator3 : Logic  AllPortsSameDT=off  OutDataTypeStr=boolean
  Logical Operator4 : Logic  AllPortsSameDT=off  OutDataTypeStr=boolean
  Logical Operator5 : Logic  Operator=NOT  AllPortsSameDT=off  OutDataTypeStr=boolean
  Logical Operator6 : Logic  Inputs=3  AllPortsSameDT=off  OutDataTypeStr=boolean
  Relational Operator2 : RelationalOperator  Operator=<  OutDataTypeStr=boolean  RndMeth=Simplest
  EGRVlv_bJamVlvClsd_DSM : Outport  Tag=%
  EGRVlv_bJamVlvOpn_DSM : Outport  Tag=%  Port=2
  wires:
  Logical Operator6/1 -> Logical Operator5/1, Logical Operator4/2
  Hysteresis_S16/1 -> Logical Operator6/2
  EGRVlv_rGovDesVal/1 -> Relational Operator2/1
  Logical Operator3/1 -> EGRVlv_bJamVlvClsd_DSM/1
  Constant17/1 -> Relational Operator2/2
  Logical Operator5/1 -> Logical Operator3/2
  Relational Operator2/1 -> Logical Operator6/3
  Constant16/1 -> Hysteresis_S16/2
  Logical Operator4/1 -> EGRVlv_bJamVlvOpn_DSM/1
  EGRVlv_stJamVlv/1 -> Logical Operator4/1, Logical Operator3/1
  EGRVlv_bGovDvtMinDeb_DSM/1 -> Logical Operator6/1
  Constant15/1 -> Hysteresis_S16/3
  EGRVlv_rAct/1 -> Hysteresis_S16/1

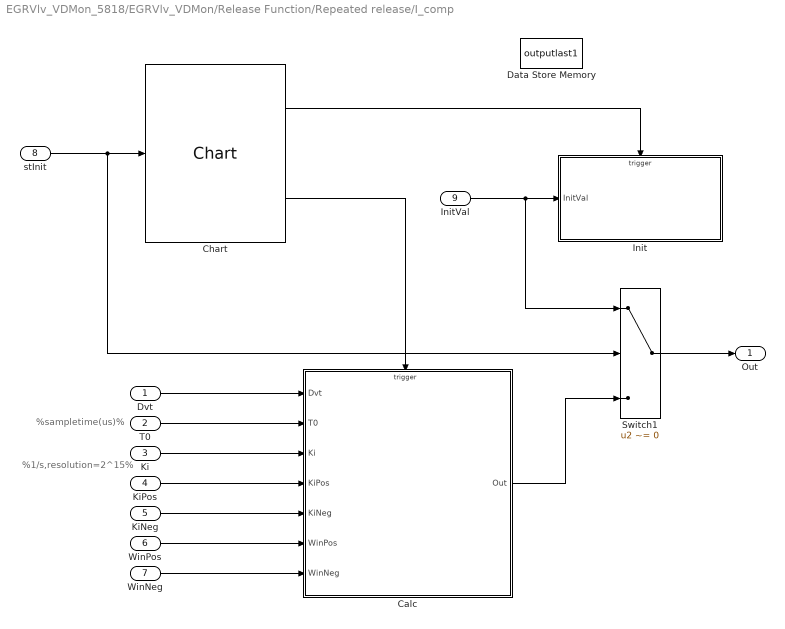
== system EGRVlv_VDMon_5818/EGRVlv_VDMon/Release Function/Repeated release/I_comp ==
  note: %sampletime(us)%
  note: %1/s,resolution=2^15%
  Dvt : Inport
  T0 : Inport  Port=2  OutDataTypeStr=uint32
  Ki : Inport  Port=3
  KiPos : Inport  Port=4
  KiNeg : Inport  Port=5
  WinPos : Inport  Port=6
  WinNeg : Inport  Port=7
  stInit : Inport  Port=8  OutDataTypeStr=boolean
  InitVal : Inport  Port=9
  Calc : Subsystem
  Chart : CXLib/I_S16/Chart
  Data Store Memory : DataStoreMemory  DataStoreName=outputlast1  ReadBeforeWriteMsg=warning  WriteAfterWriteMsg=warning  WriteAfterReadMsg=warning  ShowAdditionalParam=off  OutDataTypeStr=fixdt(1,32,2^-7,0)
  Init : Subsystem
  Switch1 : Switch  Criteria=u2 ~= 0  SaturateOnIntegerOverflow=on  InputSameDT=on
  Out : Outport
  wires:
  Chart/1 -> Init/Trigger
  stInit/1 -> Chart/1, Switch1/2
  Ki/1 -> Calc/3(Ki)
  Dvt/1 -> Calc/1(Dvt)
  T0/1 -> Calc/2(T0)
  Calc/1(Out) -> Switch1/3
  KiNeg/1 -> Calc/5(KiNeg)
  Switch1/1 -> Out/1
  Chart/2 -> Calc/Trigger
  WinNeg/1 -> Calc/7(WinNeg)
  InitVal/1 -> Init/1(InitVal), Switch1/1
  WinPos/1 -> Calc/6(WinPos)
  KiPos/1 -> Calc/4(KiPos)

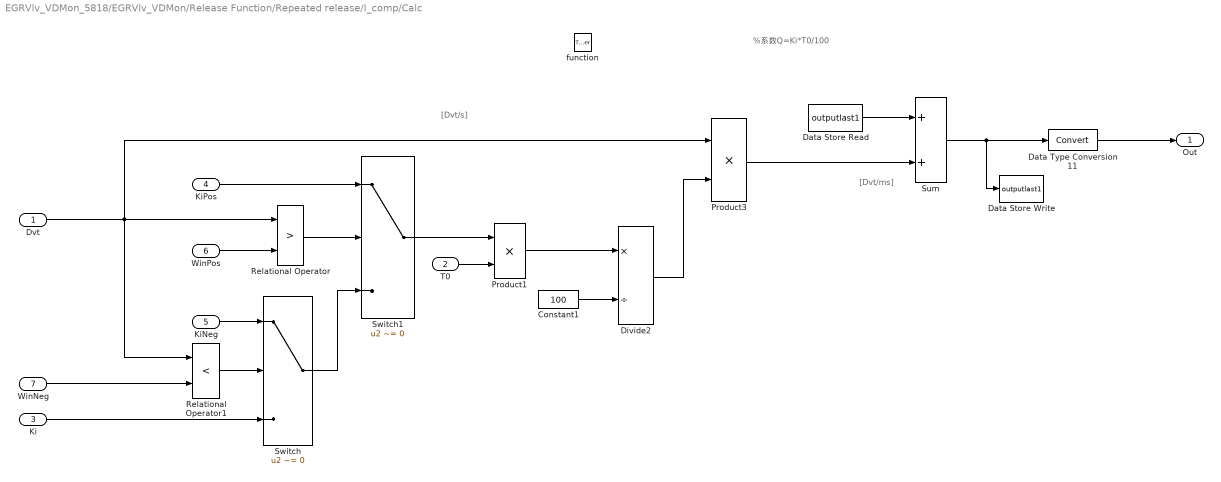
== system EGRVlv_VDMon_5818/EGRVlv_VDMon/Release Function/Repeated release/I_comp/Calc ==
  note: %系数Q=Ki*T0/100
  note: [Dvt/s]
  note: [Dvt/ms]
  Dvt : Inport
  T0 : Inport  Port=2
  Ki : Inport  Port=3
  KiPos : Inport  Port=4
  KiNeg : Inport  Port=5
  WinPos : Inport  Port=6
  WinNeg : Inport  Port=7
  function : TriggerPort  TriggerType=function-call  VariantControl=Variant
  Constant1 : Constant  Value=100  OutDataTypeStr=uint32
  Data Store Read : DataStoreRead  DataStoreName=outputlast1
  Data Store Write : DataStoreWrite  DataStoreName=outputlast1
  Data Type Conversion11 : DataTypeConversion
  Divide2 : Product  Inputs=*/  OutDataTypeStr=fixdt(1,32,2^-7,0)  RndMeth=Round  SaturateOnIntegerOverflow=on
  Product1 : Product  OutDataTypeStr=fixdt(1,32,2^-5,0)  RndMeth=Round  SaturateOnIntegerOverflow=on
  Product3 : Product  OutDataTypeStr=fixdt(1,32,2^-7,0)  RndMeth=Round  SaturateOnIntegerOverflow=on
  Relational Operator : RelationalOperator  Operator=>  OutDataTypeStr=boolean  RndMeth=Nearest  InputSameDT=on
  Relational Operator1 : RelationalOperator  Operator=<  OutDataTypeStr=boolean  RndMeth=Nearest  InputSameDT=on
  Sum : Sum  OutDataTypeStr=fixdt(1,32,2^-7,0)  RndMeth=Round  SaturateOnIntegerOverflow=on  InputSameDT=on
  Switch : Switch  Criteria=u2 ~= 0  SaturateOnIntegerOverflow=on  InputSameDT=on
  Switch1 : Switch  Criteria=u2 ~= 0  SaturateOnIntegerOverflow=on  InputSameDT=on
  Out : Outport
  wires:
  Product3/1 -> Sum/2
  Divide2/1 -> Product3/2
  Constant1/1 -> Divide2/2
  Product1/1 -> Divide2/1
  Data Type Conversion11/1 -> Out/1
  Sum/1 -> Data Type Conversion11/1, Data Store Write/1
  Dvt/1 -> Relational Operator1/1, Relational Operator/1, Product3/1
  Switch1/1 -> Product1/1
  T0/1 -> Product1/2
  WinNeg/1 -> Relational Operator1/2
  Ki/1 -> Switch/3
  Data Store Read/1 -> Sum/1
  Switch/1 -> Switch1/3
  WinPos/1 -> Relational Operator/2
  Relational Operator1/1 -> Switch/2
  KiNeg/1 -> Switch/1
  Relational Operator/1 -> Switch1/2
  KiPos/1 -> Switch1/1

== system EGRVlv_VDMon_5818/EGRVlv_VDMon/Release Function/Repeated release/I_comp/Init ==
  InitVal : Inport
  function : TriggerPort  TriggerType=function-call  VariantControl=Variant
  Constant2 : Constant  OutDataTypeStr=uint32
  Data Store Write : DataStoreWrite  DataStoreName=outputlast1
  Divide1 : Product  Inputs=**  OutDataTypeStr=Inherit: Inherit via back propagation  RndMeth=Round  SaturateOnIntegerOverflow=on
  wires:
  Constant2/1 -> Divide1/2
  Divide1/1 -> Data Store Write/1
  InitVal/1 -> Divide1/1
